simulink model "MF007_MotVltgSVPWM"  (R2022b)
settings: configuration reference "ASW_Configuration_Set_100ms" (kept outside this file)
values from neighbouring files (symbols this model uses):
  MotCtrlModeEnum : value not decoded    [XPSbW_PublicDataType.sldd]
undefined symbols (not defined in the file or in its folder): CalC_MF007_b_ManMotPwmCtrlEna_UL, CalC_MF007_f32_1D3_UL, CalC_MF007_f32_BrdgVoltFbkFilCoeff_UL, CalC_MF007_f32_ManMotPwmACmd_UL, CalC_MF007_f32_ManMotPwmBCmd_UL, CalC_MF007_f32_ManMotPwmCCmd_UL, CalC_MF007_f32_MotBrdgVltg_V, CalC_MF007_f32_MotCtrlPWMPeriodHiLimit_UL, CalC_MF007_f32_MotCtrlPWMPeriodLowLimit_UL, CalC_MF007_f32_MotPWMTimeDelay_s, CalC_MF007_f32_MotTen_UL, CalC_MF007_f32_MotThreeHundredAndFifty_UL, CalC_MF007_f32_MotZeroAgCounter_UL, CalC_MF007_f32_MotZeroAgone_UL, CalC_MF007_f32_MotZeroAgthree_UL, CalC_MF007_f32_MotZeroAgtwo_UL, CalC_MF007_f32_MoyBrdgVoltLo_V, CalC_MF007_f32_Neg1D2_UL, CalC_MF007_f32_Sqrt3D2_UL, CalC_MF007_f32_ZeroAgCalVolt_V, CalC_XPSbW_b_MotTypSeln_UL, CalC_XPSbW_b_MotZeroCalsEn_UL, Con_XPSbW_b_True_UL, Con_XPSbW_f32_1D100_UL, Con_XPSbW_f32_1D2_UL, Con_XPSbW_f32_Deg2Rad_UL, Con_XPSbW_f32_ES003MotAgArbdMax_deg, Con_XPSbW_f32_ES003MotAgArbdMin_deg, Con_XPSbW_f32_ES004MotVelElecFildMax_radps, Con_XPSbW_f32_ES004MotVelElecFildMin_radps, Con_XPSbW_f32_ES008EPSSupplyVltgMax_V, Con_XPSbW_f32_ES008EPSSupplyVltgMin_V, Con_XPSbW_f32_NegOne_UL, Con_XPSbW_f32_One_UL, Con_XPSbW_f32_Sqrt3_UL, Con_XPSbW_f32_Sqrt3D3_UL, Con_XPSbW_f32_Two_UL, Con_XPSbW_f32_Zero_UL, Con_XPSbW_u8_Four_UL, Con_XPSbW_u8_One_UL, Con_XPSbW_u8_Two_UL, Con_XPSbW_u8_Zero_UL
libraries: XpengCHASbWLib x63, simulink x4
(part 1 of 2)
settings Model: DataDictionary=MF007_MotVltgSVPWM.sldd  Creator=donglx1  LastModifiedBy=Xpeng
settings ConfigSetRef: SourceName=ASW_Configuration_Set_100ms

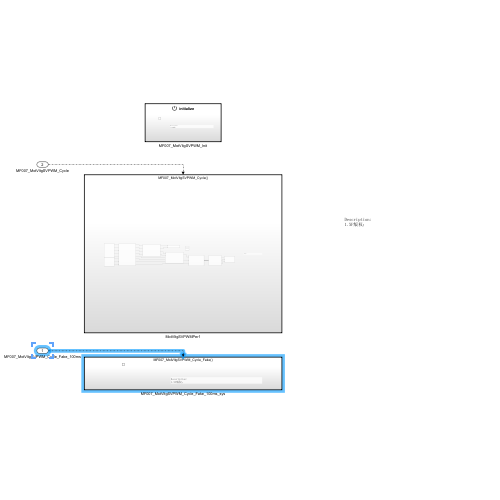
[thumbnail: Simulink's stored preview of the top-level diagram]
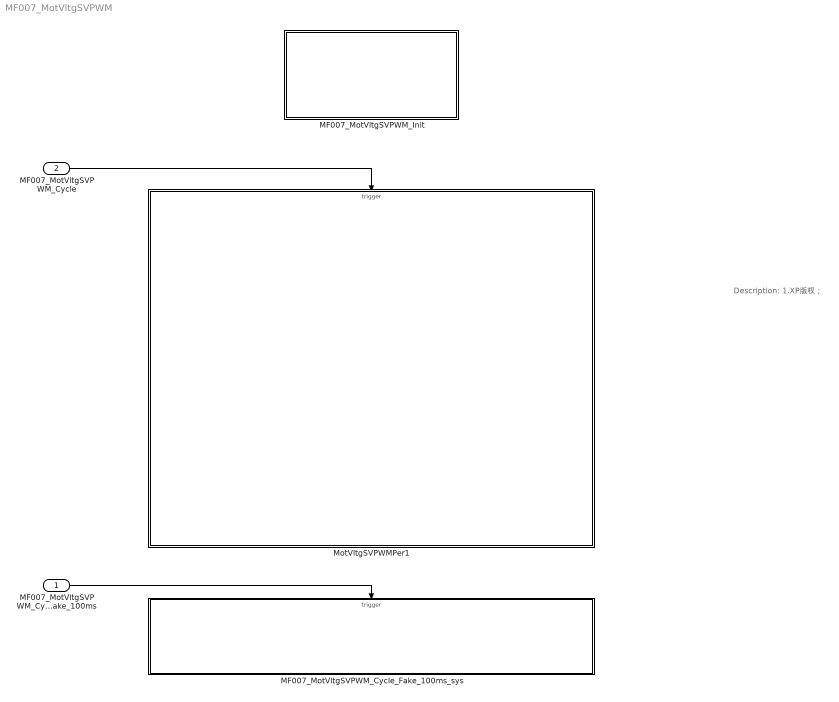
== system MF007_MotVltgSVPWM ==
  note: Description:
      | 1.XP版权；
  MF007_MotVltgSVPWM_Cycle_Fake_100ms : Inport  SampleTime=0.1  OutputFunctionCall=on
  MF007_MotVltgSVPWM_Cycle : Inport  Port=2  SampleTime=0.1  OutputFunctionCall=on
  MF007_MotVltgSVPWM_Cycle_Fake_100ms_sys : Subsystem
  MF007_MotVltgSVPWM_Init : Subsystem
  MotVltgSVPWMPer1 : Subsystem
  wires:
  MF007_MotVltgSVPWM_Cycle_Fake_100ms/1 -> MF007_MotVltgSVPWM_Cycle_Fake_100ms_sys/Trigger
  MF007_MotVltgSVPWM_Cycle/1 -> MotVltgSVPWMPer1/Trigger

== system MF007_MotVltgSVPWM/MF007_MotVltgSVPWM_Cycle_Fake_100ms_sys ==
  note: Description:
      | 1.XP版权；
  MF007_MotVltgSVPWM_Cycle_Fake : TriggerPort  TriggerType=function-call  VariantControl=(inherit)  SampleTimeType=periodic  SampleTime=-1
      settings: AttributesFormatString=|
      | SampleTimeType=%<SampleTimeType>
      | SampleTime=%<SampleTime>

== system MF007_MotVltgSVPWM/MF007_MotVltgSVPWM_Init ==
  note: Description:
      | 1.XP版权；
  MF007_MotVltgSVPWM_Init : EventListener  EventName=reset

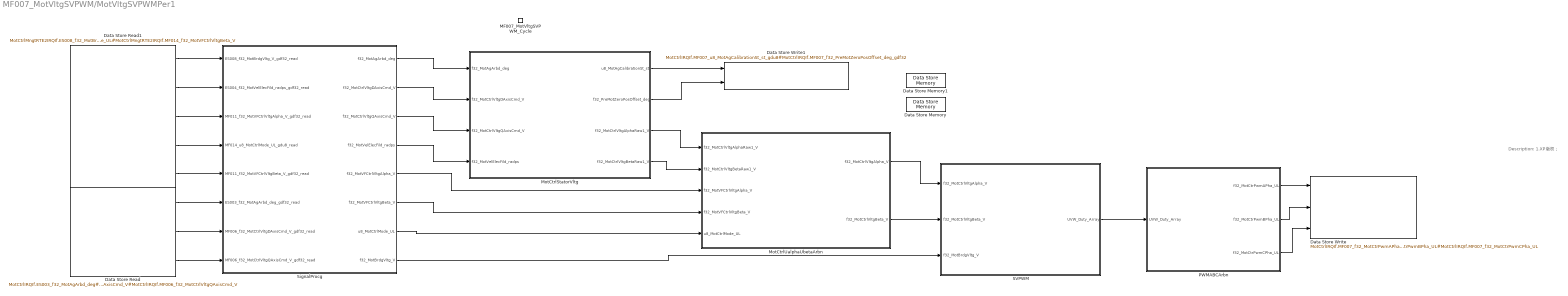
== system MF007_MotVltgSVPWM/MotVltgSVPWMPer1 ==
  note: Description:
      | 1.XP版权；
  MF007_MotVltgSVPWM_Cycle : TriggerPort  TriggerType=function-call  VariantControl=(inherit)  SampleTimeType=periodic  SampleTime=-1
      settings: AttributesFormatString=|
      | SampleTimeType=%<SampleTimeType>
      | SampleTime=%<SampleTime>
  Data Store Memory : XpengCHASbWLib/XpengCHASbWBaseLib/Signal Routing/Data Store Memory  DataStoreName=MotCtrlIRQIf  ReadBeforeWriteMsg=none  WriteAfterWriteMsg=warning  WriteAfterReadMsg=none  InitialValue=0  ShareAcrossModelInstances=off  ShowAdditionalParam=off  OutMin=[]  OutMax=[]  Dimensions=-1  StateMustResolveToSignalObject=on
      settings: SourceProductName=Xpeng CHA SbW Lib  SignalType=auto  DataLogging=off  DataLoggingLimitDataPoints=off  DataLoggingMaxPoints=5000  DataLoggingDecimateData=off  DataLoggingDecimation=2  DataLoggingNameMode=SignalName
  Data Store Memory1 : XpengCHASbWLib/XpengCHASbWBaseLib/Signal Routing/Data Store Memory  DataStoreName=MotCtrlMngtRTE2IRQIf  ReadBeforeWriteMsg=none  WriteAfterWriteMsg=warning  WriteAfterReadMsg=none  InitialValue=0  ShareAcrossModelInstances=off  ShowAdditionalParam=off  OutMin=[]  OutMax=[]  Dimensions=-1  StateMustResolveToSignalObject=on
      settings: SourceProductName=Xpeng CHA SbW Lib  SignalType=auto  DataLogging=off  DataLoggingLimitDataPoints=off  DataLoggingMaxPoints=5000  DataLoggingDecimateData=off  DataLoggingDecimation=2  DataLoggingNameMode=SignalName
  Data Store Read : DataStoreRead  DataStoreName=MotCtrlIRQIf  DataStoreElements=MotCtrlIRQIf.ES003_f32_MotAgArbd_deg#MotCtrlIRQIf.MF006_f32_MotCtrlVltgDAxisCmd_V#MotCtrlIRQIf.MF006_f32_MotCtrlVltgQAxisCmd_V  IndexOptions=Index vector (dialog)  Indices=1  OutputSizes=1
  Data Store Read1 : DataStoreRead  DataStoreName=MotCtrlMngtRTE2IRQIf  DataStoreElements=MotCtrlMngtRTE2IRQIf.ES008_f32_MotBrdgVltg_V#MotCtrlMngtRTE2IRQIf.ES004_f32_MotVelElecFild_radps#MotCtrlMngtRTE2IRQIf.MF014_f32_MotVFCtrlVltgAlpha_V#MotCtrlMngtRTE2IRQIf.MF014_u8_MotCtrlMode_UL#MotCtrlMngtRTE2IRQIf.MF014_f32_MotVFCtrlVltgBeta_V  IndexOptions=Index vector (dialog)  Indices=1  OutputSizes=1
  Data Store Write : DataStoreWrite  DataStoreName=MotCtrlIRQIf  DataStoreElements=MotCtrlIRQIf.MF007_f32_MotCtrPwmAPha_UL#MotCtrlIRQIf.MF007_f32_MotCtrPwmBPha_UL#MotCtrlIRQIf.MF007_f32_MotCtrPwmCPha_UL  IndexOptions=Index vector (dialog)  Indices=1  OutputSizes=1
  Data Store Write1 : DataStoreWrite  DataStoreName=MotCtrlIRQIf  DataStoreElements=MotCtrlIRQIf.MF007_u8_MotAgCalibrationSt_st_gdu8#MotCtrlIRQIf.MF007_f32_PreMotZeroPosOffset_deg_gdf32  IndexOptions=Index vector (dialog)  Indices=1  OutputSizes=1
  MotCtrlStatorVltg : Subsystem
  MotCtrlUalphaUbetaArbn : Subsystem
  PWMABCArbn : Subsystem
  SVPWM : Subsystem
  SignalProcg : Subsystem
  wires:
  SignalProcg/5(f32_MotVFCtrlVltgAlpha_V) -> MotCtrlUalphaUbetaArbn/3(f32_MotVFCtrlVltgAlpha_V)
  MotCtrlUalphaUbetaArbn/1(f32_MotCtrlVltgAlpha_V) -> SVPWM/1(f32_MotCtrlVltgAlpha_V)
  MotCtrlStatorVltg/3(f32_MotCtrlVltgAlphaRaw1_V) -> MotCtrlUalphaUbetaArbn/1(f32_MotCtrlVltgAlphaRaw1_V)
  SignalProcg/4(f32_MotVelElecFild_radps) -> MotCtrlStatorVltg/4(f32_MotVelElecFild_radps)
  SignalProcg/8(f32_MotBrdgVltg_V) -> SVPWM/3(f32_MotBrdgVltg_V)
  SVPWM/1(UVW_Duty_Array) -> PWMABCArbn/1(UVW_Duty_Array)
  MotCtrlStatorVltg/4(f32_MotCtrlVltgBetaRaw1_V) -> MotCtrlUalphaUbetaArbn/2(f32_MotCtrlVltgBetaRaw1_V)
  MotCtrlUalphaUbetaArbn/2(f32_MotCtrlVltgBeta_V) -> SVPWM/2(f32_MotCtrlVltgBeta_V)
  SignalProcg/2(f32_MotCtrlVltgDAxisCmd_V) -> MotCtrlStatorVltg/2(f32_MotCtrlVltgDAxisCmd_V)
  SignalProcg/7(u8_MotCtrlMode_UL) -> MotCtrlUalphaUbetaArbn/5(u8_MotCtrlMode_UL)
  SignalProcg/3(f32_MotCtrlVltgQAxisCmd_V) -> MotCtrlStatorVltg/3(f32_MotCtrlVltgQAxisCmd_V)
  SignalProcg/1(f32_MotAgArbd_deg) -> MotCtrlStatorVltg/1(f32_MotAgArbd_deg)
  SignalProcg/6(f32_MotVFCtrlVltgBeta_V) -> MotCtrlUalphaUbetaArbn/4(f32_MotVFCtrlVltgBeta_V)
  PWMABCArbn/1(f32_MotCtrPwmAPha_UL) -> Data Store Write/1
  PWMABCArbn/2(f32_MotCtrPwmBPha_UL) -> Data Store Write/2
  PWMABCArbn/3(f32_MotCtrPwmCPha_UL) -> Data Store Write/3
  Data Store Read/3 -> SignalProcg/8(MF006_f32_MotCtrlVltgQAxisCmd_V_gdf32_read)
  Data Store Read/2 -> SignalProcg/7(MF006_f32_MotCtrlVltgDAxisCmd_V_gdf32_read)
  Data Store Read/1 -> SignalProcg/6(ES003_f32_MotAgArbd_deg_gdf32_read)
  Data Store Read1/1 -> SignalProcg/1(ES008_f32_MotBrdgVltg_V_gdf32_read)
  Data Store Read1/2 -> SignalProcg/2(ES004_f32_MotVelElecFild_radps_gdf32_read)
  Data Store Read1/3 -> SignalProcg/3(MF011_f32_MotVFCtrlVltgAlpha_V_gdf32_read)
  Data Store Read1/4 -> SignalProcg/4(MF014_u8_MotCtrlMode_UL_gdu8_read)
  Data Store Read1/5 -> SignalProcg/5(MF011_f32_MotVFCtrlVltgBeta_V_gdf32_read)
  MotCtrlStatorVltg/1(u8_MotAgCalibrationSt_st) -> Data Store Write1/1
  MotCtrlStatorVltg/2(f32_PreMotZeroPosOffset_deg) -> Data Store Write1/2

== system MF007_MotVltgSVPWM/MotVltgSVPWMPer1/MotCtrlStatorVltg ==
  note: Description:
      | 1.XP版权；
  f32_MotAgArbd_deg : Inport
  f32_MotCtrlVltgDAxisCmd_V : Inport  Port=2
  f32_MotCtrlVltgQAxisCmd_V : Inport  Port=3
  f32_MotVelElecFild_radps : Inport  Port=4
  Subsystem : Subsystem
  Subsystem1 : Subsystem
  Subsystem2 : Subsystem
  Subsystem4 : Subsystem
  u8_MotAgCalibrationSt_st : Outport
      settings: EnsureOutportIsVirtual=on
  f32_PreMotZeroPosOffset_deg : Outport  Port=2
      settings: EnsureOutportIsVirtual=on
  f32_MotCtrlVltgAlphaRaw1_V : Outport  Port=3
  f32_MotCtrlVltgBetaRaw1_V : Outport  Port=4
  wires:
  f32_MotAgArbd_deg/1 -> Subsystem2/1(f32_MotAgArbd_deg), Subsystem1/1(f32_MotAgArbd_deg)
  Subsystem/1(b_MotZeroAgCalEn_flg) -> Subsystem1/Action
  Subsystem/2(b_MotZeroAgCalDisable_flg) -> Subsystem2/Action
  Subsystem1/1(u8_MotAgCalibrationSt_st) -> u8_MotAgCalibrationSt_st/1
  f32_MotCtrlVltgDAxisCmd_V/1 -> Subsystem2/2(f32_MotCtrlVltgDAxisCmd_V)
  f32_MotCtrlVltgQAxisCmd_V/1 -> Subsystem2/3(f32_MotCtrlVltgQAxisCmd_V)
  f32_MotVelElecFild_radps/1 -> Subsystem2/4(f32_MotVelElecFild_radps)
  Subsystem1/3(f32_MotZeroAgVolUalpha_V) -> Subsystem4/1(f32_MotZeroAgVolUalpha_V)
  Subsystem1/4(f32_MotZeroAgVolubeta_V) -> Subsystem4/2(f32_MotZeroAgVolubeta_V)
  Subsystem2/1(f32_MotCtrlVltgAlphaRaw_V) -> Subsystem4/3(f32_MotCtrlVltgAlphaRaw_V)
  Subsystem2/2(f32_MotCtrlVltgBetaRaw_V) -> Subsystem4/4(f32_MotCtrlVltgBetaRaw_V)
  Subsystem4/2(f32_MotCtrlVltgBetaRaw1_V) -> f32_MotCtrlVltgBetaRaw1_V/1
  Subsystem4/1(f32_MotCtrlVltgAlphaRaw1_V) -> f32_MotCtrlVltgAlphaRaw1_V/1
  Subsystem1/2(f32_PreMotZeroPosOffset_deg) -> f32_PreMotZeroPosOffset_deg/1

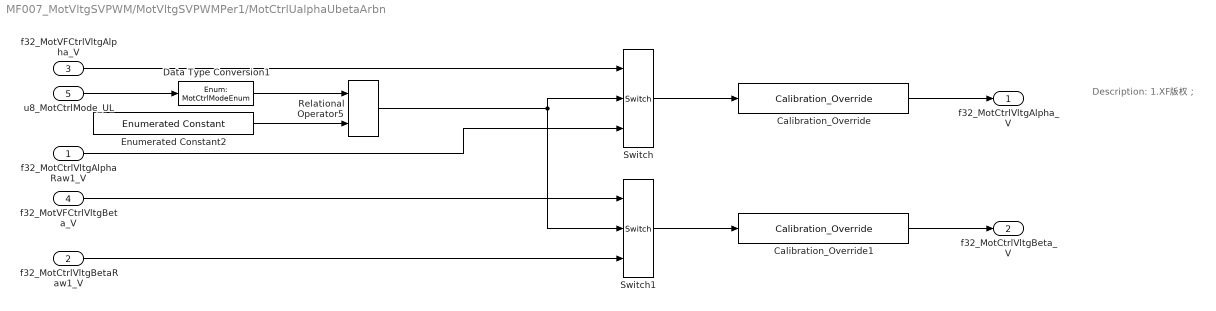
== system MF007_MotVltgSVPWM/MotVltgSVPWMPer1/MotCtrlUalphaUbetaArbn ==
  note: Description:
      | 1.XP版权；
  f32_MotCtrlVltgAlphaRaw1_V : Inport
  f32_MotCtrlVltgBetaRaw1_V : Inport  Port=2
  f32_MotVFCtrlVltgAlpha_V : Inport  Port=3
  f32_MotVFCtrlVltgBeta_V : Inport  Port=4
  u8_MotCtrlMode_UL : Inport  Port=5
  Calibration_Override : XpengCHASbWLib/XpengCHASbWAlgoLib/Signal Routing/Calibration_Override  cal_ovrdflg=CalEn_MF007_b_MotCtrlVltgUalphaEn_UL  cal_ovrdval=CalVal_MF007_f32_MotCtrlVltgUalpha_V
      settings: SourceProductName=Xpeng CHA SbW Lib
      settings: AttributesFormatString=|
      | OvrdEn:%<cal_ovrdflg>
      | OvrdVal:%<cal_ovrdval>
  Calibration_Override1 : XpengCHASbWLib/XpengCHASbWAlgoLib/Signal Routing/Calibration_Override  cal_ovrdflg=CalEn_MF007_b_MotCtrlVltgUbetaEn_UL  cal_ovrdval=CalVal_MF007_f32_MotCtrlVltgUbeta_V
      settings: SourceProductName=Xpeng CHA SbW Lib
      settings: AttributesFormatString=|
      | OvrdEn:%<cal_ovrdflg>
      | OvrdVal:%<cal_ovrdval>
  Data Type Conversion1 : DataTypeConversion  OutDataTypeStr=Enum: MotCtrlModeEnum  SaturateOnIntegerOverflow=off  RndMeth=Floor
  Enumerated Constant2 : simulink/Sources/Enumerated Constant  OutDataTypeStr=Enum: MotCtrlModeEnum  Value=MotCtrlModeEnum.VoltMod  SampleTime=inf
  Relational Operator5 : XpengCHASbWLib/XpengCHASbWBaseLib/Logic Operations/Relational Operator  Operator===  InputSameDT=on  OutDataTypeStr=Inherit: Logical (see Configuration Parameters: Optimization)  SampleTime=-1  RndMeth=Nearest
      settings: SourceProductName=Xpeng CHA SbW Lib
  Switch : XpengCHASbWLib/XpengCHASbWBaseLib/Signal Routing/Switch  Criteria=u2 ~= 0  Threshold=0  InputSameDT=on  OutMin=[]  OutMax=[]  SaturateOnIntegerOverflow=on  SampleTime=-1  AllowDiffInputSizes=off
      settings: AttributesFormatString=%<Criteria>  SourceProductName=Xpeng CHA SbW Lib
  Switch1 : XpengCHASbWLib/XpengCHASbWBaseLib/Signal Routing/Switch  Criteria=u2 ~= 0  Threshold=0  InputSameDT=on  OutMin=[]  OutMax=[]  SaturateOnIntegerOverflow=on  SampleTime=-1  AllowDiffInputSizes=off
      settings: AttributesFormatString=%<Criteria>  SourceProductName=Xpeng CHA SbW Lib
  f32_MotCtrlVltgAlpha_V : Outport
  f32_MotCtrlVltgBeta_V : Outport  Port=2
  wires:
  Switch/1 -> Calibration_Override/1
  Switch1/1 -> Calibration_Override1/1
  u8_MotCtrlMode_UL/1 -> Data Type Conversion1/1
  Enumerated Constant2/1 -> Relational Operator5/2
  Relational Operator5/1 -> Switch/2, Switch1/2
  f32_MotVFCtrlVltgBeta_V/1 -> Switch1/1
  Calibration_Override/1 -> f32_MotCtrlVltgAlpha_V/1
  Calibration_Override1/1 -> f32_MotCtrlVltgBeta_V/1
  f32_MotCtrlVltgAlphaRaw1_V/1 -> Switch/3
  f32_MotCtrlVltgBetaRaw1_V/1 -> Switch1/3
  f32_MotVFCtrlVltgAlpha_V/1 -> Switch/1
  Data Type Conversion1/1 -> Relational Operator5/1

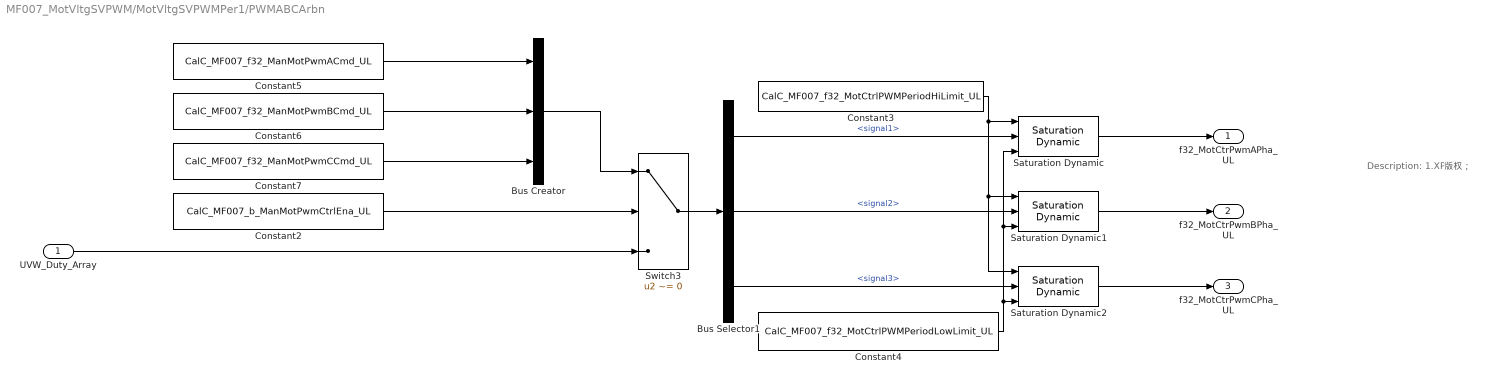
== system MF007_MotVltgSVPWM/MotVltgSVPWMPer1/PWMABCArbn ==
  note: Description:
      | 1.XP版权；
  UVW_Duty_Array : Inport
  Bus Creator : BusCreator  Inputs=3
  Bus Selector1 : BusSelector  OutputSignals=signal1,signal2,signal3
  Constant2 : Constant  Value=CalC_MF007_b_ManMotPwmCtrlEna_UL
  Constant3 : Constant  Value=CalC_MF007_f32_MotCtrlPWMPeriodHiLimit_UL
  Constant4 : Constant  Value=CalC_MF007_f32_MotCtrlPWMPeriodLowLimit_UL
  Constant5 : Constant  Value=CalC_MF007_f32_ManMotPwmACmd_UL
  Constant6 : Constant  Value=CalC_MF007_f32_ManMotPwmBCmd_UL
  Constant7 : Constant  Value=CalC_MF007_f32_ManMotPwmCCmd_UL
  Saturation Dynamic : simulink/Discontinuities/Saturation Dynamic  OutMin=[]  OutMax=[]  OutDataTypeStr=Inherit: Same as second input  OutDataType=fixdt(1, 16)  OutScaling=2^-10  DoSatur=off
  Saturation Dynamic1 : simulink/Discontinuities/Saturation Dynamic  OutMin=[]  OutMax=[]  OutDataTypeStr=Inherit: Same as second input  OutDataType=fixdt(1, 16)  OutScaling=2^-10  DoSatur=off
  Saturation Dynamic2 : simulink/Discontinuities/Saturation Dynamic  OutMin=[]  OutMax=[]  OutDataTypeStr=Inherit: Same as second input  OutDataType=fixdt(1, 16)  OutScaling=2^-10  DoSatur=off
  Switch3 : Switch  Criteria=u2 ~= 0  SaturateOnIntegerOverflow=off  InputSameDT=off
  f32_MotCtrPwmAPha_UL : Outport
      settings: EnsureOutportIsVirtual=on
  f32_MotCtrPwmBPha_UL : Outport  Port=2
      settings: EnsureOutportIsVirtual=on
  f32_MotCtrPwmCPha_UL : Outport  Port=3
      settings: EnsureOutportIsVirtual=on
  wires:
  Switch3/1 -> Bus Selector1/1
  Constant3/1 -> Saturation Dynamic2/1, Saturation Dynamic1/1, Saturation Dynamic/1
  Saturation Dynamic1/1 -> f32_MotCtrPwmBPha_UL/1
  Constant4/1 -> Saturation Dynamic/3, Saturation Dynamic1/3, Saturation Dynamic2/3
  Saturation Dynamic/1 -> f32_MotCtrPwmAPha_UL/1
  Bus Selector1/3 -> Saturation Dynamic2/2  "<signal3>"
  UVW_Duty_Array/1 -> Switch3/3
  Saturation Dynamic2/1 -> f32_MotCtrPwmCPha_UL/1
  Constant5/1 -> Bus Creator/1
  Bus Selector1/1 -> Saturation Dynamic/2  "<signal1>"
  Constant7/1 -> Bus Creator/3
  Bus Selector1/2 -> Saturation Dynamic1/2  "<signal2>"
  Constant2/1 -> Switch3/2
  Constant6/1 -> Bus Creator/2
  Bus Creator/1 -> Switch3/1

== system MF007_MotVltgSVPWM/MotVltgSVPWMPer1/SVPWM ==
  note: Description:
      | 1.XP版权；
  f32_MotCtrlVltgAlpha_V : Inport
  f32_MotCtrlVltgBeta_V : Inport  Port=2
  f32_MotBrdgVltg_V : Inport  Port=3
  OvermodulationProcg : Subsystem
  SectorCal : Subsystem
  XYZ : Subsystem
  XYZ1 : Subsystem
  XYZ2 : Subsystem
  UVW_Duty_Array : Outport  VectorParamsAs1DForOutWhenUnconnected=off
  wires:
  f32_MotCtrlVltgBeta_V/1 -> XYZ/2(f32_MotCtrlVltgBeta_V), SectorCal/2(f32_MotCtrlVltgBeta_V)
  f32_MotCtrlVltgAlpha_V/1 -> XYZ/1(f32_MotCtrlVltgAlpha_V), SectorCal/1(f32_MotCtrlVltgAlpha_V)
  f32_MotBrdgVltg_V/1 -> XYZ/3(f32_MotBrdgVltg_V)
  XYZ/3(Z) -> XYZ1/4(Z)
  XYZ/2(Y) -> XYZ1/3(Y)
  OvermodulationProcg/1(T12_Procg) -> XYZ2/2(T12)
  XYZ/1(X) -> XYZ1/2(X)
  SectorCal/1(u8_MotSector_UL) -> XYZ2/1(u8_MotSector_UL), XYZ1/1(u8_MotSector_UL)
  XYZ2/1(UVW_Duty_Array) -> UVW_Duty_Array/1
  XYZ1/1(T12) -> OvermodulationProcg/1(T12)

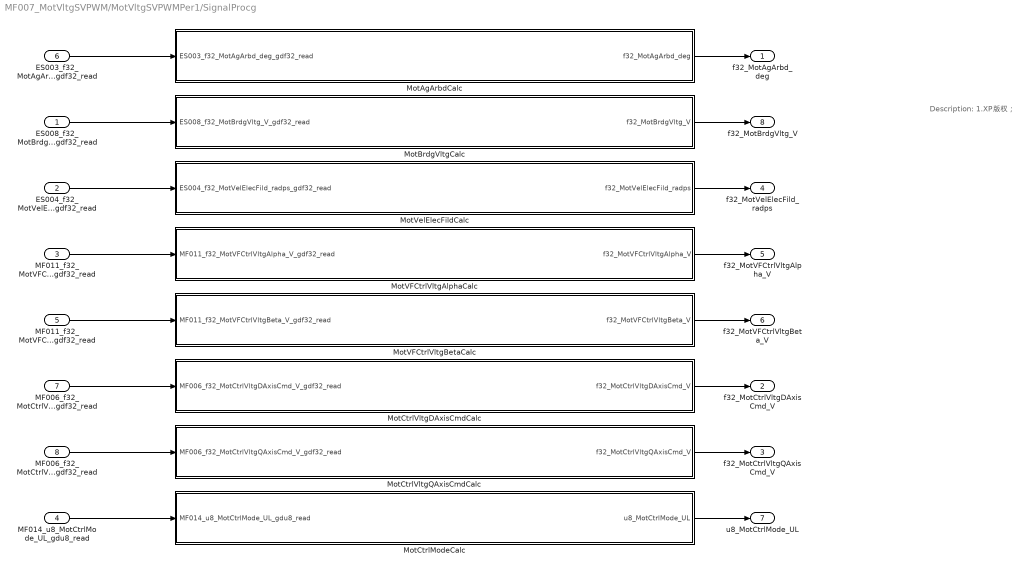
== system MF007_MotVltgSVPWM/MotVltgSVPWMPer1/SignalProcg ==
  note: Description:
      | 1.XP版权；
  ES008_f32_MotBrdgVltg_V_gdf32_read : Inport
  ES004_f32_MotVelElecFild_radps_gdf32_read : Inport  Port=2
  MF011_f32_MotVFCtrlVltgAlpha_V_gdf32_read : Inport  Port=3
  MF014_u8_MotCtrlMode_UL_gdu8_read : Inport  Port=4
  MF011_f32_MotVFCtrlVltgBeta_V_gdf32_read : Inport  Port=5
  ES003_f32_MotAgArbd_deg_gdf32_read : Inport  Port=6
  MF006_f32_MotCtrlVltgDAxisCmd_V_gdf32_read : Inport  Port=7
  MF006_f32_MotCtrlVltgQAxisCmd_V_gdf32_read : Inport  Port=8
  MotAgArbdCalc : Subsystem
  MotBrdgVltgCalc : Subsystem
  MotCtrlModeCalc : Subsystem
  MotCtrlVltgDAxisCmdCalc : Subsystem
  MotCtrlVltgQAxisCmdCalc : Subsystem
  MotVFCtrlVltgAlphaCalc : Subsystem
  MotVFCtrlVltgBetaCalc : Subsystem
  MotVelElecFildCalc : Subsystem
  f32_MotAgArbd_deg : Outport
  f32_MotCtrlVltgDAxisCmd_V : Outport  Port=2
  f32_MotCtrlVltgQAxisCmd_V : Outport  Port=3
  f32_MotVelElecFild_radps : Outport  Port=4
  f32_MotVFCtrlVltgAlpha_V : Outport  Port=5
  f32_MotVFCtrlVltgBeta_V : Outport  Port=6
  u8_MotCtrlMode_UL : Outport  Port=7
  f32_MotBrdgVltg_V : Outport  Port=8
  wires:
  ES004_f32_MotVelElecFild_radps_gdf32_read/1 -> MotVelElecFildCalc/1(ES004_f32_MotVelElecFild_radps_gdf32_read)
  ES008_f32_MotBrdgVltg_V_gdf32_read/1 -> MotBrdgVltgCalc/1(ES008_f32_MotBrdgVltg_V_gdf32_read)
  ES003_f32_MotAgArbd_deg_gdf32_read/1 -> MotAgArbdCalc/1(ES003_f32_MotAgArbd_deg_gdf32_read)
  MotAgArbdCalc/1(f32_MotAgArbd_deg) -> f32_MotAgArbd_deg/1
  MotBrdgVltgCalc/1(f32_MotBrdgVltg_V) -> f32_MotBrdgVltg_V/1
  MotVelElecFildCalc/1(f32_MotVelElecFild_radps) -> f32_MotVelElecFild_radps/1
  MF011_f32_MotVFCtrlVltgAlpha_V_gdf32_read/1 -> MotVFCtrlVltgAlphaCalc/1(MF011_f32_MotVFCtrlVltgAlpha_V_gdf32_read)
  MotVFCtrlVltgAlphaCalc/1(f32_MotVFCtrlVltgAlpha_V) -> f32_MotVFCtrlVltgAlpha_V/1
  MF011_f32_MotVFCtrlVltgBeta_V_gdf32_read/1 -> MotVFCtrlVltgBetaCalc/1(MF011_f32_MotVFCtrlVltgBeta_V_gdf32_read)
  MF006_f32_MotCtrlVltgDAxisCmd_V_gdf32_read/1 -> MotCtrlVltgDAxisCmdCalc/1(MF006_f32_MotCtrlVltgDAxisCmd_V_gdf32_read)
  MF006_f32_MotCtrlVltgQAxisCmd_V_gdf32_read/1 -> MotCtrlVltgQAxisCmdCalc/1(MF006_f32_MotCtrlVltgQAxisCmd_V_gdf32_read)
  MF014_u8_MotCtrlMode_UL_gdu8_read/1 -> MotCtrlModeCalc/1(MF014_u8_MotCtrlMode_UL_gdu8_read)
  MotVFCtrlVltgBetaCalc/1(f32_MotVFCtrlVltgBeta_V) -> f32_MotVFCtrlVltgBeta_V/1
  MotCtrlVltgDAxisCmdCalc/1(f32_MotCtrlVltgDAxisCmd_V) -> f32_MotCtrlVltgDAxisCmd_V/1
  MotCtrlVltgQAxisCmdCalc/1(f32_MotCtrlVltgQAxisCmd_V) -> f32_MotCtrlVltgQAxisCmd_V/1
  MotCtrlModeCalc/1(u8_MotCtrlMode_UL) -> u8_MotCtrlMode_UL/1

== system MF007_MotVltgSVPWM/MotVltgSVPWMPer1/MotCtrlStatorVltg/Subsystem ==
  note: Description:
      | 1.XP版权；
  Constant : Constant  Value=CalC_XPSbW_b_MotZeroCalsEn_UL
  If : If  IfExpression=u1 == 1
  b_MotZeroAgCalEn_flg : Outport
  b_MotZeroAgCalDisable_flg : Outport  Port=2
  wires:
  Constant/1 -> If/1
  If/2 -> b_MotZeroAgCalDisable_flg/1
  If/1 -> b_MotZeroAgCalEn_flg/1

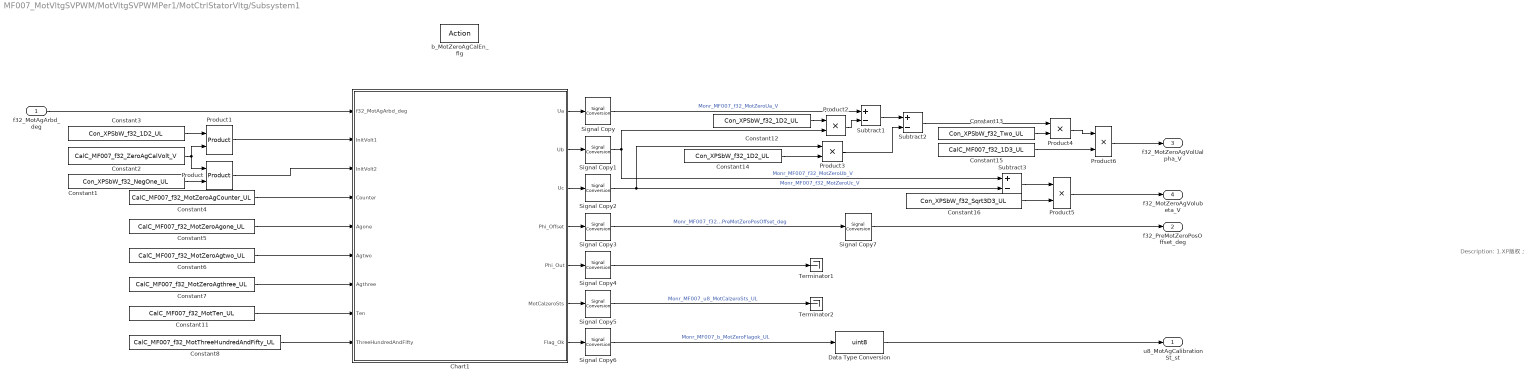
== system MF007_MotVltgSVPWM/MotVltgSVPWMPer1/MotCtrlStatorVltg/Subsystem1 ==
  note: Description:
      | 1.XP版权；
  f32_MotAgArbd_deg : Inport
  b_MotZeroAgCalEn_flg : ActionPort  ActionPortLabel=if(u1 == 1)
  Chart1 : Stateflow chart  TreatAsAtomicUnit=on
      settings: PortSchema="{\"entries\":[{\"content\":{\"sides\":[{\"content\":{\"connectorIds\":[\"In1\",\"In2\",\"In3\",\"In4\",\"In5\",\"In7\",\"In6\",\"In8\",\"In9\"]},\"type\":\"ConnectorPlacement.EquallySpacedRectSide\",\"uuid\":\"c0b776fd-f9c3-46a3-bcf2-78277c181056\"},{\"content\":{\"connectorIds\":[\"Out1\",\"Out2\",\"Out3\",\"Out4\",\"Out6\",\"Out7\",\"Out5\"],\"side\":\"RIGHT\"},\"type\":\"ConnectorPlacement.EquallySpacedRectSide\",\"uuid\":\"faec2a9b-d18f-4659-a1ec-eeaa302fe436\"},{\"content\":{\"connectorIds\":[],\"side\":\"TOP\"},\"type\":\"ConnectorPlacement.EquallySpacedRectSide\",\"uuid\":\"ae3a4ef0-e647-4d80-9ccb-63a892ad0e59\"}]},\"type\":\"ConnectorPlacement.EquallySpacedConnector\",\"uuid\":\"88ddbb7a-b53a-4e2b-831c-a44bbab1e19b\"}],\"packageUris\":[\"http://schema.mathworks.com/mf0/Connector/R2020b\"],\"version\":\"1.0\"}"
  Constant1 : Constant  Value=Con_XPSbW_f32_NegOne_UL
  Constant11 : Constant  Value=CalC_MF007_f32_MotTen_UL
  Constant12 : Constant  Value=Con_XPSbW_f32_1D2_UL  OutDataTypeStr=single
  Constant13 : Constant  Value=Con_XPSbW_f32_Two_UL  OutDataTypeStr=single
  Constant14 : Constant  Value=Con_XPSbW_f32_1D2_UL  OutDataTypeStr=single
  Constant15 : Constant  Value=CalC_MF007_f32_1D3_UL  OutDataTypeStr=single
  Constant16 : Constant  Value=Con_XPSbW_f32_Sqrt3D3_UL
  Constant2 : Constant  Value=CalC_MF007_f32_ZeroAgCalVolt_V  OutDataTypeStr=single
  Constant3 : Constant  Value=Con_XPSbW_f32_1D2_UL
  Constant4 : Constant  Value=CalC_MF007_f32_MotZeroAgCounter_UL
  Constant5 : Constant  Value=CalC_MF007_f32_MotZeroAgone_UL
  Constant6 : Constant  Value=CalC_MF007_f32_MotZeroAgtwo_UL
  Constant7 : Constant  Value=CalC_MF007_f32_MotZeroAgthree_UL
  Constant8 : Constant  Value=CalC_MF007_f32_MotThreeHundredAndFifty_UL
  Data Type Conversion : DataTypeConversion  OutDataTypeStr=uint8  SaturateOnIntegerOverflow=off  RndMeth=Floor
  Product : XpengCHASbWLib/XpengCHASbWBaseLib/Math Operations/Product  Inputs=2  Multiplication=Element-wise(.*)  CollapseDim=1  OutMin=[]  OutMax=[]  RndMeth=Zero  SaturateOnIntegerOverflow=on  SampleTime=-1
      settings: SourceProductName=Xpeng CHA SbW Lib
  Product1 : XpengCHASbWLib/XpengCHASbWBaseLib/Math Operations/Product  Inputs=2  Multiplication=Element-wise(.*)  CollapseDim=1  OutMin=[]  OutMax=[]  RndMeth=Zero  SaturateOnIntegerOverflow=on  SampleTime=-1
      settings: SourceProductName=Xpeng CHA SbW Lib
  Product{2..6} (5 alike) : Product
  Signal Copy{,1..7} (8 alike) : SignalConversion  OverrideOpt=off
  Subtract1 : Sum  Inputs=+-
  Subtract2 : Sum  Inputs=+-
  Subtract3 : Sum  Inputs=+-
  Terminator1 : Terminator
  Terminator2 : Terminator
  u8_MotAgCalibrationSt_st : Outport
  f32_PreMotZeroPosOffset_deg : Outport  Port=2
      settings: EnsureOutportIsVirtual=on
  f32_MotZeroAgVolUalpha_V : Outport  Port=3  VectorParamsAs1DForOutWhenUnconnected=off
  f32_MotZeroAgVolubeta_V : Outport  Port=4  VectorParamsAs1DForOutWhenUnconnected=off
  wires:
  Constant7/1 -> Chart1/6(Agthree)
  Product1/1 -> Chart1/2(InitVolt1)
  Constant1/1 -> Product/2
  Chart1/1(Ua) -> Signal Copy/1
  Constant4/1 -> Chart1/4(Counter)
  Constant6/1 -> Chart1/7(Agtwo)
  Signal Copy2/1 -> Subtract3/2, Product3/1  "Monr_MF007_f32_MotZeroUc_V"
  Constant2/1 -> Product/1, Product1/2
  Product/1 -> Chart1/3(InitVolt2)
  Constant5/1 -> Chart1/5(Agone)
  f32_MotAgArbd_deg/1 -> Chart1/1(f32_MotAgArbd_deg)
  Constant3/1 -> Product1/1
  Signal Copy3/1 -> Signal Copy7/1  "Monr_MF007_f32_PreMotZeroPosOffset_deg"
  Signal Copy1/1 -> Product2/2, Subtract3/1  "Monr_MF007_f32_MotZeroUb_V"
  Product6/1 -> f32_MotZeroAgVolUalpha_V/1
  Product5/1 -> f32_MotZeroAgVolubeta_V/1
  Signal Copy6/1 -> Data Type Conversion/1  "Monr_MF007_b_MotZeroFlagok_UL"
  Data Type Conversion/1 -> u8_MotAgCalibrationSt_st/1
  Constant11/1 -> Chart1/8(Ten)
  Constant12/1 -> Product2/1
  Product2/1 -> Subtract1/2
  Constant14/1 -> Product3/2
  Subtract1/1 -> Subtract2/1
  Product3/1 -> Subtract2/2
  Subtract2/1 -> Product4/1
  Constant13/1 -> Product4/2
  Product4/1 -> Product6/1
  Constant15/1 -> Product6/2
  Constant16/1 -> Product5/2
  Subtract3/1 -> Product5/1
  Signal Copy5/1 -> Terminator2/1  "Monr_MF007_u8_MotCalzeroSts_UL"
  Signal Copy/1 -> Subtract1/1  "Monr_MF007_f32_MotZeroUa_V"
  Chart1/2(Ub) -> Signal Copy1/1
  Chart1/3(Uc) -> Signal Copy2/1
  Chart1/4(Phi_Offset) -> Signal Copy3/1
  Chart1/7(MotCalzeroSts) -> Signal Copy5/1
  Chart1/6(Phi_Out) -> Signal Copy4/1
  Chart1/5(Flag_Ok) -> Signal Copy6/1
  Signal Copy7/1 -> f32_PreMotZeroPosOffset_deg/1
  Constant8/1 -> Chart1/9(ThreeHundredAndFifty)
  Signal Copy4/1 -> Terminator1/1

== system MF007_MotVltgSVPWM/MotVltgSVPWMPer1/MotCtrlStatorVltg/Subsystem2 ==
  note: Description:
      | 1.XP版权；
  f32_MotAgArbd_deg : Inport
  f32_MotCtrlVltgDAxisCmd_V : Inport  Port=2
  f32_MotCtrlVltgQAxisCmd_V : Inport  Port=3
  f32_MotVelElecFild_radps : Inport  Port=4
  b_MotZeroAgCalDisable_flg : ActionPort  ActionPortLabel=else
  Subsystem : Subsystem
  Subsystem1 : Subsystem
  Subsystem2 : Subsystem
  Subsystem3 : Subsystem
  Subsystem4 : Subsystem
  f32_MotCtrlVltgAlphaRaw_V : Outport
  f32_MotCtrlVltgBetaRaw_V : Outport  Port=2
  wires:
  f32_MotAgArbd_deg/1 -> Subsystem/1(f32_MotAgArbd_deg)
  f32_MotCtrlVltgDAxisCmd_V/1 -> Subsystem/2(f32_MotCtrlVltgDAxisCmd_V)
  f32_MotCtrlVltgQAxisCmd_V/1 -> Subsystem/3(f32_MotCtrlVltgQAxisCmd_V)
  f32_MotVelElecFild_radps/1 -> Subsystem/4(f32_MotVelElecFild_radps)
  Subsystem/1(f32_MotCtrlVltgAlpha_V) -> Subsystem3/1(f32_MotCtrlVltgAlphaRaw_V), Subsystem2/1(f32_MotCtrlVltgAlphaRaw_V)
  Subsystem/2(f32_MotCtrlVltgBeta_V) -> Subsystem2/2(f32_MotCtrlVltgBetaRaw_V), Subsystem3/2(f32_MotCtrlVltgBetaRaw_V)
  Subsystem1/1(StarMotor) -> Subsystem2/Action
  Subsystem1/2(DeltaMotor) -> Subsystem3/Action
  Subsystem2/1(f32_StarMotCtrlVltgAlpha_V) -> Subsystem4/1(f32_StarMotCtrlVltgAlpha_V)
  Subsystem2/2(f32_StarMotCtrlVltgBeta_V) -> Subsystem4/2(f32_StarMotCtrlVltgBeta_V)
  Subsystem3/1(f32_DeltaMotCtrlVltgAlpha_V) -> Subsystem4/3(f32_DeltaMotCtrlVltgAlpha_V)
  Subsystem3/2(f32_DeltaMotCtrlVltgBeta_V) -> Subsystem4/4(f32_DeltaMotCtrlVltgBeta_V)
  Subsystem4/1(f32_MotCtrlVltgAlphaRaw_V) -> f32_MotCtrlVltgAlphaRaw_V/1
  Subsystem4/2(f32_MotCtrlVltgBetaRaw_V) -> f32_MotCtrlVltgBetaRaw_V/1

== system MF007_MotVltgSVPWM/MotVltgSVPWMPer1/MotCtrlStatorVltg/Subsystem4 ==
  note: Description:
      | 1.XP版权；
  f32_MotZeroAgVolUalpha_V : Inport
  f32_MotZeroAgVolubeta_V : Inport  Port=2
  f32_MotCtrlVltgAlphaRaw_V : Inport  Port=3
  f32_MotCtrlVltgBetaRaw_V : Inport  Port=4
  Merge : Merge
  Merge1 : Merge
  f32_MotCtrlVltgAlphaRaw1_V : Outport
  f32_MotCtrlVltgBetaRaw1_V : Outport  Port=2
  wires:
  f32_MotZeroAgVolUalpha_V/1 -> Merge/1
  f32_MotCtrlVltgAlphaRaw_V/1 -> Merge/2
  Merge/1 -> f32_MotCtrlVltgAlphaRaw1_V/1
  f32_MotZeroAgVolubeta_V/1 -> Merge1/1
  f32_MotCtrlVltgBetaRaw_V/1 -> Merge1/2
  Merge1/1 -> f32_MotCtrlVltgBetaRaw1_V/1

== system MF007_MotVltgSVPWM/MotVltgSVPWMPer1/SVPWM/OvermodulationProcg ==
  note: Description:
      | 1.XP版权；
  T12 : Inport
  Add : Sum
  Bus Creator6 : BusCreator  Inputs=2
  Bus Selector : BusSelector  OutputSignals=signal1,signal2
  Constant1 : Constant  Value=Con_XPSbW_f32_One_UL
  DIV : XpengCHASbWLib/XpengCHASbWBaseLib/Math Operations/DIV  MinRange=single(1e-6)
      settings: SourceProductName=Xpeng CHA SbW Lib
  DIV1 : XpengCHASbWLib/XpengCHASbWBaseLib/Math Operations/DIV  MinRange=single(1e-6)
      settings: SourceProductName=Xpeng CHA SbW Lib
  Relational Operator : RelationalOperator  Operator=>  RndMeth=Simplest  InputSameDT=off
  Switch : XpengCHASbWLib/XpengCHASbWBaseLib/Signal Routing/Switch  Criteria=u2 ~= 0  Threshold=0  InputSameDT=on  OutMin=[]  OutMax=[]  SaturateOnIntegerOverflow=on  SampleTime=-1  AllowDiffInputSizes=off
      settings: AttributesFormatString=%<Criteria>  SourceProductName=Xpeng CHA SbW Lib
  T12_Procg : Outport
  wires:
  DIV1/1 -> Bus Creator6/2
  Bus Creator6/1 -> Switch/1
  Add/1 -> DIV/2, DIV1/2, Relational Operator/1
  T12/1 -> Bus Selector/1, Switch/3
  Bus Selector/2 -> Add/2, DIV1/1  "<signal2>"
  DIV/1 -> Bus Creator6/1
  Bus Selector/1 -> Add/1, DIV/1  "<signal1>"
  Switch/1 -> T12_Procg/1
  Constant1/1 -> Relational Operator/2
  Relational Operator/1 -> Switch/2

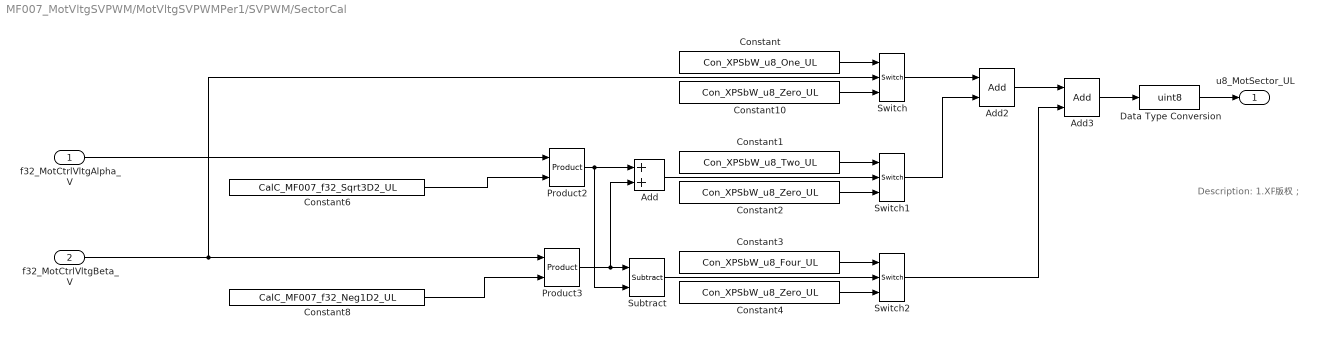
== system MF007_MotVltgSVPWM/MotVltgSVPWMPer1/SVPWM/SectorCal ==
  note: Description:
      | 1.XP版权；
  f32_MotCtrlVltgAlpha_V : Inport
  f32_MotCtrlVltgBeta_V : Inport  Port=2
  Add : Sum
  Add2 : XpengCHASbWLib/XpengCHASbWBaseLib/Math Operations/Add  Inputs=++  CollapseDim=1  OutMin=[]  OutMax=[]  SampleTime=-1
      settings: SourceProductName=Xpeng CHA SbW Lib
  Add3 : XpengCHASbWLib/XpengCHASbWBaseLib/Math Operations/Add  Inputs=++  CollapseDim=1  OutMin=[]  OutMax=[]  SampleTime=-1
      settings: SourceProductName=Xpeng CHA SbW Lib
  Constant : Constant  Value=Con_XPSbW_u8_One_UL  OutDataTypeStr=single
  Constant1 : Constant  Value=Con_XPSbW_u8_Two_UL  OutDataTypeStr=single
  Constant10 : Constant  Value=Con_XPSbW_u8_Zero_UL  OutDataTypeStr=single
  Constant2 : Constant  Value=Con_XPSbW_u8_Zero_UL  OutDataTypeStr=single
  Constant3 : Constant  Value=Con_XPSbW_u8_Four_UL  OutDataTypeStr=single
  Constant4 : Constant  Value=Con_XPSbW_u8_Zero_UL  OutDataTypeStr=single
  Constant6 : Constant  Value=CalC_MF007_f32_Sqrt3D2_UL
  Constant8 : Constant  Value=CalC_MF007_f32_Neg1D2_UL
  Data Type Conversion : DataTypeConversion  OutDataTypeStr=uint8  SaturateOnIntegerOverflow=off  RndMeth=Floor
  Product2 : XpengCHASbWLib/XpengCHASbWBaseLib/Math Operations/Product  Inputs=2  Multiplication=Element-wise(.*)  CollapseDim=1  OutMin=[]  OutMax=[]  RndMeth=Zero  SaturateOnIntegerOverflow=on  SampleTime=-1
      settings: SourceProductName=Xpeng CHA SbW Lib
  Product3 : XpengCHASbWLib/XpengCHASbWBaseLib/Math Operations/Product  Inputs=2  Multiplication=Element-wise(.*)  CollapseDim=1  OutMin=[]  OutMax=[]  RndMeth=Zero  SaturateOnIntegerOverflow=on  SampleTime=-1
      settings: SourceProductName=Xpeng CHA SbW Lib
  Subtract : XpengCHASbWLib/XpengCHASbWBaseLib/Math Operations/Subtract  Inputs=+-  CollapseDim=1  OutMin=[]  OutMax=[]  SampleTime=-1
      settings: SourceProductName=Xpeng CHA SbW Lib
  Switch : XpengCHASbWLib/XpengCHASbWBaseLib/Signal Routing/Switch  Criteria=u2 > Threshold  Threshold=0  InputSameDT=on  OutMin=[]  OutMax=[]  SaturateOnIntegerOverflow=on  SampleTime=-1  AllowDiffInputSizes=off
      settings: AttributesFormatString=%<Criteria>  SourceProductName=Xpeng CHA SbW Lib
  Switch1 : XpengCHASbWLib/XpengCHASbWBaseLib/Signal Routing/Switch  Criteria=u2 > Threshold  Threshold=0  InputSameDT=on  OutMin=[]  OutMax=[]  SaturateOnIntegerOverflow=on  SampleTime=-1  AllowDiffInputSizes=off
      settings: AttributesFormatString=%<Criteria>  SourceProductName=Xpeng CHA SbW Lib
  Switch2 : XpengCHASbWLib/XpengCHASbWBaseLib/Signal Routing/Switch  Criteria=u2 > Threshold  Threshold=0  InputSameDT=on  OutMin=[]  OutMax=[]  SaturateOnIntegerOverflow=on  SampleTime=-1  AllowDiffInputSizes=off
      settings: AttributesFormatString=%<Criteria>  SourceProductName=Xpeng CHA SbW Lib
  u8_MotSector_UL : Outport
  wires:
  Constant/1 -> Switch/1
  f32_MotCtrlVltgAlpha_V/1 -> Product2/1
  Constant10/1 -> Switch/3
  f32_MotCtrlVltgBeta_V/1 -> Switch/2, Product3/1
  Product2/1 -> Subtract/2, Add/1
  Product3/1 -> Add/2, Subtract/1
  Constant1/1 -> Switch1/1
  Constant2/1 -> Switch1/3
  Add/1 -> Switch1/2
  Constant3/1 -> Switch2/1
  Subtract/1 -> Switch2/2
  Add3/1 -> Data Type Conversion/1
  Constant6/1 -> Product2/2
  Constant8/1 -> Product3/2
  Constant4/1 -> Switch2/3
  Switch/1 -> Add2/1
  Switch1/1 -> Add2/2
  Add2/1 -> Add3/1
  Switch2/1 -> Add3/2
  Data Type Conversion/1 -> u8_MotSector_UL/1

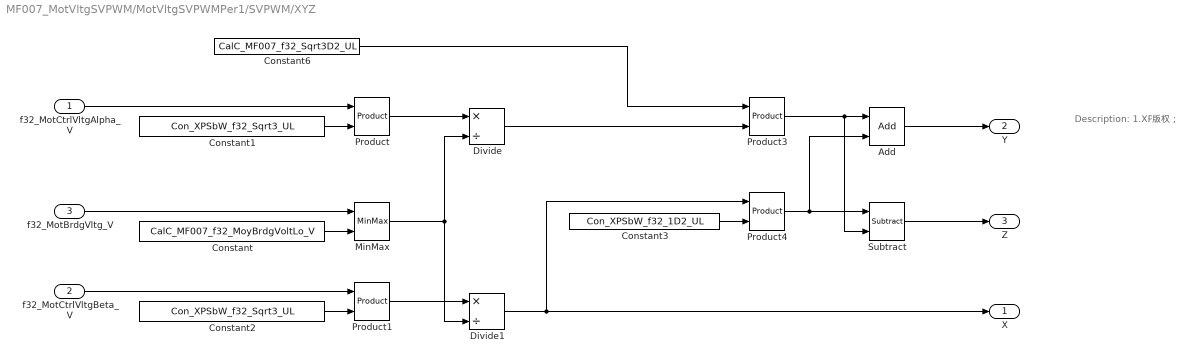
== system MF007_MotVltgSVPWM/MotVltgSVPWMPer1/SVPWM/XYZ ==
  note: Description:
      | 1.XP版权；
  f32_MotCtrlVltgAlpha_V : Inport
  f32_MotCtrlVltgBeta_V : Inport  Port=2
  f32_MotBrdgVltg_V : Inport  Port=3
  Add : XpengCHASbWLib/XpengCHASbWBaseLib/Math Operations/Add  Inputs=++  CollapseDim=1  OutMin=[]  OutMax=[]  SampleTime=-1
      settings: SourceProductName=Xpeng CHA SbW Lib
  Constant : Constant  Value=CalC_MF007_f32_MoyBrdgVoltLo_V  OutDataTypeStr=single
  Constant1 : Constant  Value=Con_XPSbW_f32_Sqrt3_UL  OutDataTypeStr=single
  Constant2 : Constant  Value=Con_XPSbW_f32_Sqrt3_UL  OutDataTypeStr=single
  Constant3 : Constant  Value=Con_XPSbW_f32_1D2_UL
  Constant6 : Constant  Value=CalC_MF007_f32_Sqrt3D2_UL
  Divide : Product  Inputs=*/
  Divide1 : Product  Inputs=*/
  MinMax : XpengCHASbWLib/XpengCHASbWBaseLib/Math Operations/MinMax  Function=max  Inputs=2  InputSameDT=on  OutMin=[]  OutMax=[]  SaturateOnIntegerOverflow=on  SampleTime=-1
      settings: SourceProductName=Xpeng CHA SbW Lib
  Product{,1,3..4} (4 alike) : XpengCHASbWLib/XpengCHASbWBaseLib/Math Operations/Product  Inputs=2  Multiplication=Element-wise(.*)  CollapseDim=1  OutMin=[]  OutMax=[]  RndMeth=Zero  SaturateOnIntegerOverflow=on  SampleTime=-1
      settings: SourceProductName=Xpeng CHA SbW Lib
  Subtract : XpengCHASbWLib/XpengCHASbWBaseLib/Math Operations/Subtract  Inputs=+-  CollapseDim=1  OutMin=[]  OutMax=[]  SampleTime=-1
      settings: SourceProductName=Xpeng CHA SbW Lib
  X : Outport
  Y : Outport  Port=2
  Z : Outport  Port=3
  wires:
  f32_MotCtrlVltgAlpha_V/1 -> Product/1
  Product/1 -> Divide/1
  f32_MotBrdgVltg_V/1 -> MinMax/1
  f32_MotCtrlVltgBeta_V/1 -> Product1/1
  Product1/1 -> Divide1/1
  Divide1/1 -> X/1, Product4/1
  Divide/1 -> Product3/2
  Product3/1 -> Add/1, Subtract/2
  Product4/1 -> Add/2, Subtract/1
  Add/1 -> Y/1
  Subtract/1 -> Z/1
  MinMax/1 -> Divide1/2, Divide/2
  Constant/1 -> MinMax/2
  Constant1/1 -> Product/2
  Constant2/1 -> Product1/2
  Constant6/1 -> Product3/1
  Constant3/1 -> Product4/2

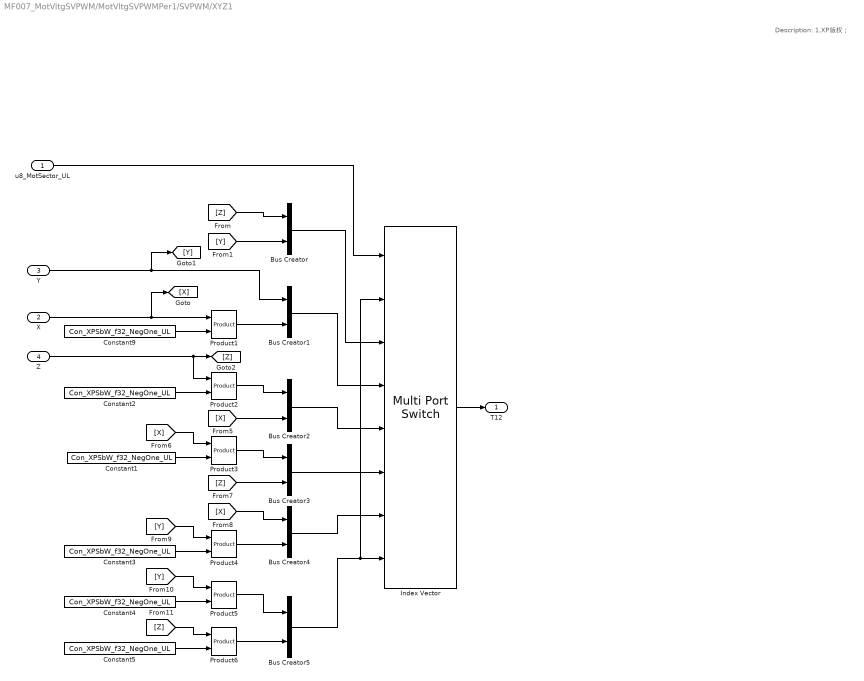
== system MF007_MotVltgSVPWM/MotVltgSVPWMPer1/SVPWM/XYZ1 ==
  note: Description:
      | 1.XP版权；
  u8_MotSector_UL : Inport
  X : Inport  Port=2
  Y : Inport  Port=3
  Z : Inport  Port=4
  Bus Creator{,1..5} (6 alike) : BusCreator  Inputs=2
  Constant{1..5,9} (6 alike) : Constant  Value=Con_XPSbW_f32_NegOne_UL
  Index Vector : MultiPortSwitch  DataPortOrder=Zero-based contiguous  Inputs=7  DataPortIndices={1,2,3,4,5,6}  DiagnosticForDefault=None  zeroidx=on  SaturateOnIntegerOverflow=off  InputSameDT=off
  Product{1..6} (6 alike) : XpengCHASbWLib/XpengCHASbWBaseLib/Math Operations/Product  Inputs=2  Multiplication=Element-wise(.*)  CollapseDim=1  OutMin=[]  OutMax=[]  RndMeth=Zero  SaturateOnIntegerOverflow=on  SampleTime=-1
      settings: SourceProductName=Xpeng CHA SbW Lib
  T12 : Outport
  wires:
  Index Vector/1 -> T12/1
  X/1 -> Product1/1, [X]
  Constant3/1 -> Product4/2
  [Z] -> Bus Creator3/2
  Constant2/1 -> Product2/2
  Constant1/1 -> Product3/2
  Constant9/1 -> Product1/2
  [X] -> Product3/1
  Z/1 -> [Z], Product2/1
  [Y] -> Product4/1
  Y/1 -> Bus Creator1/1, [Y]
  [Y] -> Product5/1
  [X] -> Bus Creator2/2
  [Z] -> Product6/1
  Constant4/1 -> Product5/2
  Constant5/1 -> Product6/2
  [Z] -> Bus Creator/1
  [Y] -> Bus Creator/2
  Product1/1 -> Bus Creator1/2
  Product2/1 -> Bus Creator2/1
  Product3/1 -> Bus Creator3/1
  [X] -> Bus Creator4/1
  Product6/1 -> Bus Creator5/2
  Product4/1 -> Bus Creator4/2
  Product5/1 -> Bus Creator5/1
  u8_MotSector_UL/1 -> Index Vector/1
  Bus Creator/1 -> Index Vector/3
  Bus Creator1/1 -> Index Vector/4
  Bus Creator2/1 -> Index Vector/5
  Bus Creator3/1 -> Index Vector/6
  Bus Creator4/1 -> Index Vector/7
  Bus Creator5/1 -> Index Vector/2, Index Vector/8

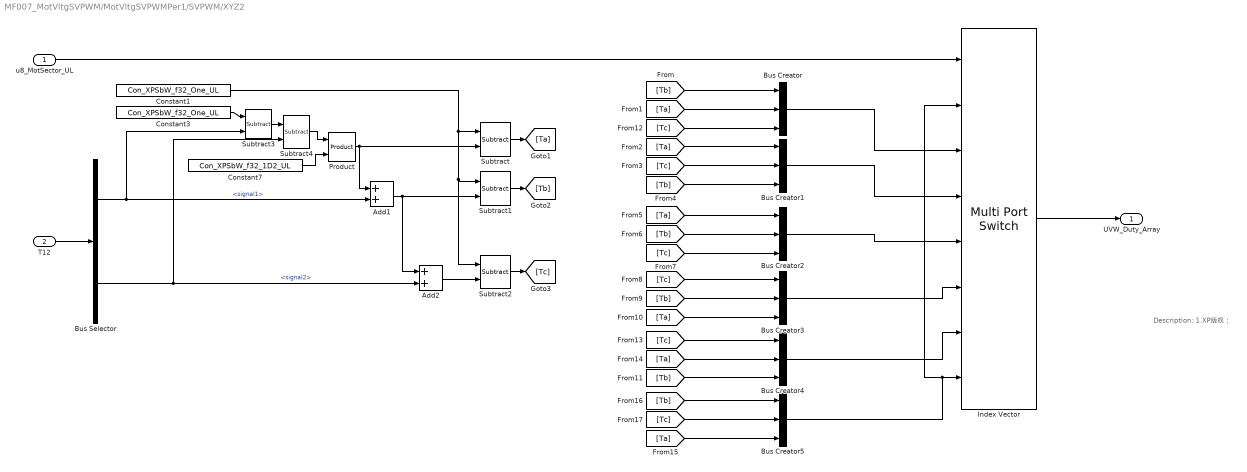
== system MF007_MotVltgSVPWM/MotVltgSVPWMPer1/SVPWM/XYZ2 ==
  note: Description:
      | 1.XP版权；
  u8_MotSector_UL : Inport
  T12 : Inport  Port=2
  Add1 : Sum
  Add2 : Sum
  Bus Creator{,1..5} (6 alike) : BusCreator  Inputs=3
  Bus Selector : BusSelector  OutputSignals=signal1,signal2
  Constant1 : Constant  Value=Con_XPSbW_f32_One_UL
  Constant3 : Constant  Value=Con_XPSbW_f32_One_UL
  Constant7 : Constant  Value=Con_XPSbW_f32_1D2_UL
  Index Vector : MultiPortSwitch  DataPortOrder=Zero-based contiguous  Inputs=7  DataPortIndices={1,2,3,4,5,6}  DiagnosticForDefault=None  zeroidx=on  SaturateOnIntegerOverflow=off  InputSameDT=off
  Product : XpengCHASbWLib/XpengCHASbWBaseLib/Math Operations/Product  Inputs=2  Multiplication=Element-wise(.*)  CollapseDim=1  OutMin=[]  OutMax=[]  RndMeth=Zero  SaturateOnIntegerOverflow=on  SampleTime=-1
      settings: SourceProductName=Xpeng CHA SbW Lib
  Subtract{,1..4} (5 alike) : XpengCHASbWLib/XpengCHASbWBaseLib/Math Operations/Subtract  Inputs=+-  CollapseDim=1  OutMin=[]  OutMax=[]  SampleTime=-1
      settings: SourceProductName=Xpeng CHA SbW Lib
  UVW_Duty_Array : Outport
  wires:
  Index Vector/1 -> UVW_Duty_Array/1
  [Ta] -> Bus Creator/2
  [Tb] -> Bus Creator/1
  u8_MotSector_UL/1 -> Index Vector/1
  [Tc] -> Bus Creator/3
  [Tc] -> Bus Creator1/2
  [Ta] -> Bus Creator1/1
  [Tb] -> Bus Creator1/3
  [Tb] -> Bus Creator2/2
  [Ta] -> Bus Creator2/1
  [Tc] -> Bus Creator2/3
  [Tb] -> Bus Creator3/2
  [Tc] -> Bus Creator3/1
  [Ta] -> Bus Creator3/3
  [Ta] -> Bus Creator4/2
  [Tc] -> Bus Creator4/1
  [Tb] -> Bus Creator4/3
  [Tc] -> Bus Creator5/2
  [Tb] -> Bus Creator5/1
  [Ta] -> Bus Creator5/3
  Add1/1 -> Subtract1/2, Add2/1
  T12/1 -> Bus Selector/1
  Bus Selector/2 -> Subtract4/2, Add2/2  "<signal2>"
  Constant3/1 -> Subtract3/1
  Subtract2/1 -> [Tc]
  Subtract3/1 -> Subtract4/1
  Bus Selector/1 -> Add1/2, Subtract3/2  "<signal1>"
  Product/1 -> Subtract/2, Add1/1
  Constant1/1 -> Subtract1/1, Subtract2/1, Subtract/1
  Subtract/1 -> [Ta]
  Add2/1 -> Subtract2/2
  Subtract1/1 -> [Tb]
  Constant7/1 -> Product/2
  Subtract4/1 -> Product/1
  Bus Creator/1 -> Index Vector/3
  Bus Creator1/1 -> Index Vector/4
  Bus Creator2/1 -> Index Vector/5
  Bus Creator3/1 -> Index Vector/6
  Bus Creator4/1 -> Index Vector/7
  Bus Creator5/1 -> Index Vector/2, Index Vector/8

== system MF007_MotVltgSVPWM/MotVltgSVPWMPer1/SignalProcg/MotAgArbdCalc ==
  note: Description:
      | 1.XP版权；
  ES003_f32_MotAgArbd_deg_gdf32_read : Inport
  Constant : Constant  Value=Con_XPSbW_f32_ES003MotAgArbdMax_deg
  Constant1 : Constant  Value=Con_XPSbW_f32_ES003MotAgArbdMin_deg
  Constant2 : Constant  Value=Con_XPSbW_f32_1D100_UL
  Constant3 : Constant  Value=Con_XPSbW_f32_Zero_UL
  Signal Copy3 : SignalConversion  OverrideOpt=off
  SignalValidityJudgementFloat4 : XpengCHASbWLib/XpengCHASbWAlgoLib/Diagnostic/SignalValidityJudgementFloat
      settings: SourceProductName=Xpeng CHA SbW Lib
  Switch : XpengCHASbWLib/XpengCHASbWBaseLib/Signal Routing/Switch  Criteria=u2 ~= 0  Threshold=0  InputSameDT=on  OutMin=[]  OutMax=[]  SaturateOnIntegerOverflow=on  SampleTime=-1  AllowDiffInputSizes=off
      settings: AttributesFormatString=%<Criteria>  SourceProductName=Xpeng CHA SbW Lib
  f32_MotAgArbd_deg : Outport
  wires:
  Constant1/1 -> SignalValidityJudgementFloat4/3
  ES003_f32_MotAgArbd_deg_gdf32_read/1 -> Signal Copy3/1, SignalValidityJudgementFloat4/1
  Constant2/1 -> SignalValidityJudgementFloat4/4
  Switch/1 -> f32_MotAgArbd_deg/1
  Signal Copy3/1 -> Switch/1
  SignalValidityJudgementFloat4/1 -> Switch/2
  Constant3/1 -> Switch/3
  Constant/1 -> SignalValidityJudgementFloat4/2

== system MF007_MotVltgSVPWM/MotVltgSVPWMPer1/SignalProcg/MotBrdgVltgCalc ==
  note: Description:
      | 1.XP版权；
  ES008_f32_MotBrdgVltg_V_gdf32_read : Inport
  Constant : Constant  Value=Con_XPSbW_f32_ES008EPSSupplyVltgMax_V
  Constant1 : Constant  Value=Con_XPSbW_f32_ES008EPSSupplyVltgMin_V
  Constant10 : Constant  Value=Con_XPSbW_b_True_UL  OutDataTypeStr=single
  Constant2 : Constant  Value=Con_XPSbW_f32_1D100_UL
  Constant3 : Constant  Value=CalC_MF007_f32_MotBrdgVltg_V
  Constant9 : Constant  Value=CalC_MF007_f32_BrdgVoltFbkFilCoeff_UL  OutDataTypeStr=single
  LPF_1stOrder_TypeK : XpengCHASbWLib/XpengCHASbWAlgoLib/Digital Filters/LPF_1stOrder_TypeK
      settings: SourceProductName=Xpeng CHA SbW Lib
  Signal Copy3 : SignalConversion  OverrideOpt=off
  SignalValidityJudgementFloat4 : XpengCHASbWLib/XpengCHASbWAlgoLib/Diagnostic/SignalValidityJudgementFloat
      settings: SourceProductName=Xpeng CHA SbW Lib
  Switch : XpengCHASbWLib/XpengCHASbWBaseLib/Signal Routing/Switch  Criteria=u2 ~= 0  Threshold=0  InputSameDT=on  OutMin=[]  OutMax=[]  SaturateOnIntegerOverflow=on  SampleTime=-1  AllowDiffInputSizes=off
      settings: AttributesFormatString=%<Criteria>  SourceProductName=Xpeng CHA SbW Lib
  f32_MotBrdgVltg_V : Outport
  wires:
  Constant1/1 -> SignalValidityJudgementFloat4/3
  ES008_f32_MotBrdgVltg_V_gdf32_read/1 -> Signal Copy3/1, SignalValidityJudgementFloat4/1
  Constant2/1 -> SignalValidityJudgementFloat4/4
  LPF_1stOrder_TypeK/1 -> f32_MotBrdgVltg_V/1
  Signal Copy3/1 -> Switch/1
  SignalValidityJudgementFloat4/1 -> Switch/2
  Constant3/1 -> Switch/3
  Constant/1 -> SignalValidityJudgementFloat4/2
  Constant10/1 -> LPF_1stOrder_TypeK/3
  Constant9/1 -> LPF_1stOrder_TypeK/2
  Switch/1 -> LPF_1stOrder_TypeK/1

== system MF007_MotVltgSVPWM/MotVltgSVPWMPer1/SignalProcg/MotCtrlModeCalc ==
  note: Description:
      | 1.XP版权；
  MF014_u8_MotCtrlMode_UL_gdu8_read : Inport
  Signal Copy6 : SignalConversion  OverrideOpt=off
  u8_MotCtrlMode_UL : Outport
  wires:
  Signal Copy6/1 -> u8_MotCtrlMode_UL/1
  MF014_u8_MotCtrlMode_UL_gdu8_read/1 -> Signal Copy6/1

== system MF007_MotVltgSVPWM/MotVltgSVPWMPer1/SignalProcg/MotCtrlVltgDAxisCmdCalc ==
  note: Description:
      | 1.XP版权；
  MF006_f32_MotCtrlVltgDAxisCmd_V_gdf32_read : Inport
  Signal Copy6 : SignalConversion  OverrideOpt=off
  f32_MotCtrlVltgDAxisCmd_V : Outport
  wires:
  Signal Copy6/1 -> f32_MotCtrlVltgDAxisCmd_V/1
  MF006_f32_MotCtrlVltgDAxisCmd_V_gdf32_read/1 -> Signal Copy6/1

== system MF007_MotVltgSVPWM/MotVltgSVPWMPer1/SignalProcg/MotCtrlVltgQAxisCmdCalc ==
  note: Description:
      | 1.XP版权；
  MF006_f32_MotCtrlVltgQAxisCmd_V_gdf32_read : Inport
  Signal Copy6 : SignalConversion  OverrideOpt=off
  f32_MotCtrlVltgQAxisCmd_V : Outport
  wires:
  Signal Copy6/1 -> f32_MotCtrlVltgQAxisCmd_V/1
  MF006_f32_MotCtrlVltgQAxisCmd_V_gdf32_read/1 -> Signal Copy6/1

== system MF007_MotVltgSVPWM/MotVltgSVPWMPer1/SignalProcg/MotVFCtrlVltgAlphaCalc ==
  note: Description:
      | 1.XP版权；
  MF011_f32_MotVFCtrlVltgAlpha_V_gdf32_read : Inport
  Signal Copy6 : SignalConversion  OverrideOpt=off
  f32_MotVFCtrlVltgAlpha_V : Outport
  wires:
  Signal Copy6/1 -> f32_MotVFCtrlVltgAlpha_V/1
  MF011_f32_MotVFCtrlVltgAlpha_V_gdf32_read/1 -> Signal Copy6/1

== system MF007_MotVltgSVPWM/MotVltgSVPWMPer1/SignalProcg/MotVFCtrlVltgBetaCalc ==
  note: Description:
      | 1.XP版权；
  MF011_f32_MotVFCtrlVltgBeta_V_gdf32_read : Inport
  Signal Copy6 : SignalConversion  OverrideOpt=off
  f32_MotVFCtrlVltgBeta_V : Outport
  wires:
  Signal Copy6/1 -> f32_MotVFCtrlVltgBeta_V/1
  MF011_f32_MotVFCtrlVltgBeta_V_gdf32_read/1 -> Signal Copy6/1

== system MF007_MotVltgSVPWM/MotVltgSVPWMPer1/SignalProcg/MotVelElecFildCalc ==
  note: Description:
      | 1.XP版权；
  ES004_f32_MotVelElecFild_radps_gdf32_read : Inport
  Constant4 : Constant  Value=Con_XPSbW_f32_ES004MotVelElecFildMax_radps
  Constant5 : Constant  Value=Con_XPSbW_f32_ES004MotVelElecFildMin_radps
  Constant6 : Constant  Value=Con_XPSbW_f32_1D100_UL
  Constant7 : Constant  Value=Con_XPSbW_f32_Zero_UL
  Signal Copy6 : SignalConversion  OverrideOpt=off
  SignalValidityJudgementFloat1 : XpengCHASbWLib/XpengCHASbWAlgoLib/Diagnostic/SignalValidityJudgementFloat
      settings: SourceProductName=Xpeng CHA SbW Lib
  Switch1 : XpengCHASbWLib/XpengCHASbWBaseLib/Signal Routing/Switch  Criteria=u2 ~= 0  Threshold=0  InputSameDT=on  OutMin=[]  OutMax=[]  SaturateOnIntegerOverflow=on  SampleTime=-1  AllowDiffInputSizes=off
      settings: AttributesFormatString=%<Criteria>  SourceProductName=Xpeng CHA SbW Lib
  f32_MotVelElecFild_radps : Outport
  wires:
  Constant6/1 -> SignalValidityJudgementFloat1/4
  Switch1/1 -> f32_MotVelElecFild_radps/1
  Constant7/1 -> Switch1/3
  ES004_f32_MotVelElecFild_radps_gdf32_read/1 -> Signal Copy6/1, SignalValidityJudgementFloat1/1
  Signal Copy6/1 -> Switch1/1
  Constant5/1 -> SignalValidityJudgementFloat1/3
  SignalValidityJudgementFloat1/1 -> Switch1/2
  Constant4/1 -> SignalValidityJudgementFloat1/2

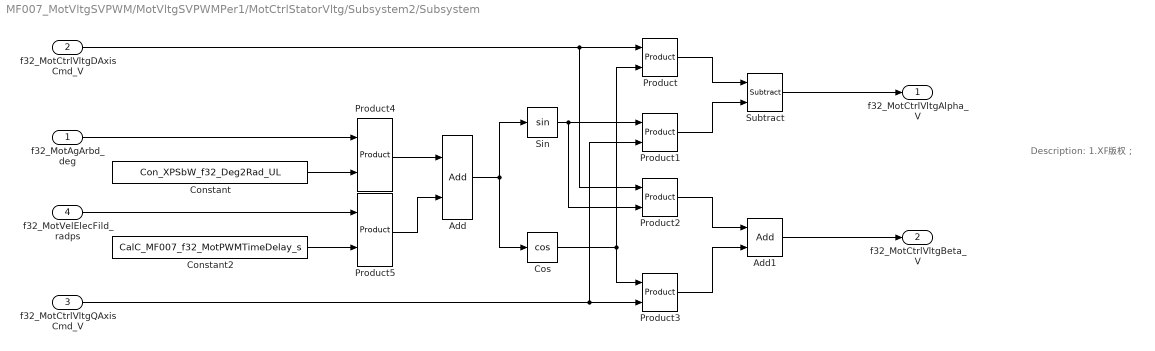
== system MF007_MotVltgSVPWM/MotVltgSVPWMPer1/MotCtrlStatorVltg/Subsystem2/Subsystem ==
  note: Description:
      | 1.XP版权；
  f32_MotAgArbd_deg : Inport
  f32_MotCtrlVltgDAxisCmd_V : Inport  Port=2
  f32_MotCtrlVltgQAxisCmd_V : Inport  Port=3
  f32_MotVelElecFild_radps : Inport  Port=4
  Add : XpengCHASbWLib/XpengCHASbWBaseLib/Math Operations/Add  Inputs=++  CollapseDim=1  OutMin=[]  OutMax=[]  SampleTime=-1
      settings: SourceProductName=Xpeng CHA SbW Lib
  Add1 : XpengCHASbWLib/XpengCHASbWBaseLib/Math Operations/Add  Inputs=++  CollapseDim=1  OutMin=[]  OutMax=[]  SampleTime=-1
      settings: SourceProductName=Xpeng CHA SbW Lib
  Constant : Constant  Value=Con_XPSbW_f32_Deg2Rad_UL
  Constant2 : Constant  Value=CalC_MF007_f32_MotPWMTimeDelay_s
  Cos : Trigonometry  Operator=cos
  Product{,1..5} (6 alike) : XpengCHASbWLib/XpengCHASbWBaseLib/Math Operations/Product  Inputs=2  Multiplication=Element-wise(.*)  CollapseDim=1  OutMin=[]  OutMax=[]  RndMeth=Zero  SaturateOnIntegerOverflow=on  SampleTime=-1
      settings: SourceProductName=Xpeng CHA SbW Lib
  Sin : Trigonometry
  Subtract : XpengCHASbWLib/XpengCHASbWBaseLib/Math Operations/Subtract  Inputs=+-  CollapseDim=1  OutMin=[]  OutMax=[]  SampleTime=-1
      settings: SourceProductName=Xpeng CHA SbW Lib
  f32_MotCtrlVltgAlpha_V : Outport
  f32_MotCtrlVltgBeta_V : Outport  Port=2
  wires:
  Product2/1 -> Add1/1
  f32_MotCtrlVltgQAxisCmd_V/1 -> Product1/2, Product3/2
  Product1/1 -> Subtract/2
  Product3/1 -> Add1/2
  Subtract/1 -> f32_MotCtrlVltgAlpha_V/1
  f32_MotCtrlVltgDAxisCmd_V/1 -> Product2/1, Product/1
  Cos/1 -> Product3/1, Product/2
  Product/1 -> Subtract/1
  Constant/1 -> Product4/2
  f32_MotVelElecFild_radps/1 -> Product5/1
  Add/1 -> Sin/1, Cos/1
  Product5/1 -> Add/2
  Sin/1 -> Product1/1, Product2/2
  f32_MotAgArbd_deg/1 -> Product4/1
  Add1/1 -> f32_MotCtrlVltgBeta_V/1
  Product4/1 -> Add/1
  Constant2/1 -> Product5/2

== system MF007_MotVltgSVPWM/MotVltgSVPWMPer1/MotCtrlStatorVltg/Subsystem2/Subsystem1 ==
  note: Description:
      | 1.XP版权；
  Constant18 : Constant  Value=CalC_XPSbW_b_MotTypSeln_UL
  If1 : XpengCHASbWLib/XpengCHASbWBaseLib/Ports&Subsystems/If  NumInputs=1  IfExpression=u1 == 0  ShowElse=on  SampleTime=-1
      settings: SourceProductName=Xpeng CHA SbW Lib
  StarMotor : Outport
  DeltaMotor : Outport  Port=2
  wires:
  Constant18/1 -> If1/1
  If1/1 -> StarMotor/1
  If1/2 -> DeltaMotor/1

== system MF007_MotVltgSVPWM/MotVltgSVPWMPer1/MotCtrlStatorVltg/Subsystem2/Subsystem2 ==
  note: Description:
      | 1.XP版权；
  f32_MotCtrlVltgAlphaRaw_V : Inport
  f32_MotCtrlVltgBetaRaw_V : Inport  Port=2
  StarMotor : ActionPort  ActionPortLabel=if(u1 == 0)
  Signal Copy : SignalConversion  OverrideOpt=off
  Signal Copy1 : SignalConversion  OverrideOpt=off
  f32_StarMotCtrlVltgAlpha_V : Outport
  f32_StarMotCtrlVltgBeta_V : Outport  Port=2
  wires:
  f32_MotCtrlVltgAlphaRaw_V/1 -> Signal Copy/1
  f32_MotCtrlVltgBetaRaw_V/1 -> Signal Copy1/1
  Signal Copy/1 -> f32_StarMotCtrlVltgAlpha_V/1
  Signal Copy1/1 -> f32_StarMotCtrlVltgBeta_V/1

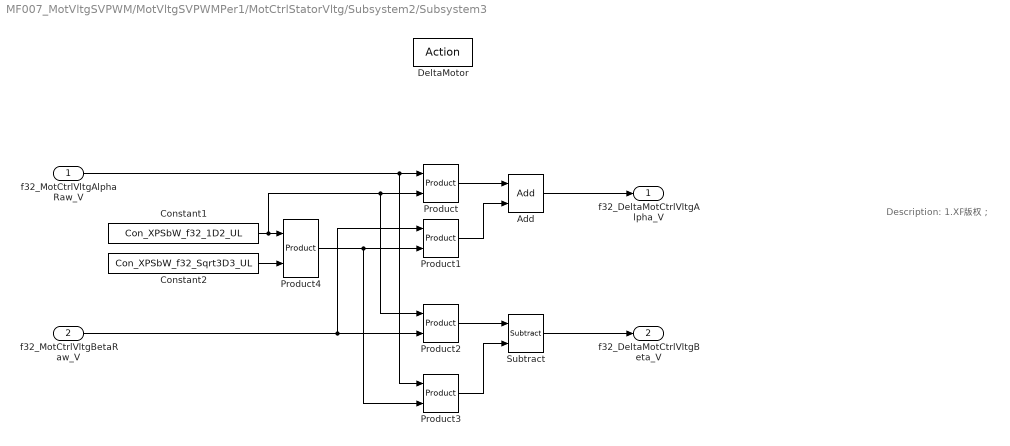
== system MF007_MotVltgSVPWM/MotVltgSVPWMPer1/MotCtrlStatorVltg/Subsystem2/Subsystem3 ==
  note: Description:
      | 1.XP版权；
  f32_MotCtrlVltgAlphaRaw_V : Inport
  f32_MotCtrlVltgBetaRaw_V : Inport  Port=2
  DeltaMotor : ActionPort  ActionPortLabel=else
  Add : XpengCHASbWLib/XpengCHASbWBaseLib/Math Operations/Add  Inputs=++  CollapseDim=1  OutMin=[]  OutMax=[]  SampleTime=-1
      settings: SourceProductName=Xpeng CHA SbW Lib
  Constant1 : Constant  Value=Con_XPSbW_f32_1D2_UL  OutDataTypeStr=single
  Constant2 : Constant  Value=Con_XPSbW_f32_Sqrt3D3_UL  OutDataTypeStr=single
  Product{,1..4} (5 alike) : XpengCHASbWLib/XpengCHASbWBaseLib/Math Operations/Product  Inputs=2  Multiplication=Element-wise(.*)  CollapseDim=1  OutMin=[]  OutMax=[]  RndMeth=Zero  SaturateOnIntegerOverflow=on  SampleTime=-1
      settings: SourceProductName=Xpeng CHA SbW Lib
  Subtract : XpengCHASbWLib/XpengCHASbWBaseLib/Math Operations/Subtract  Inputs=+-  CollapseDim=1  OutMin=[]  OutMax=[]  SampleTime=-1
      settings: SourceProductName=Xpeng CHA SbW Lib
  f32_DeltaMotCtrlVltgAlpha_V : Outport
  f32_DeltaMotCtrlVltgBeta_V : Outport  Port=2
  wires:
  f32_MotCtrlVltgAlphaRaw_V/1 -> Product3/1, Product/1
  Subtract/1 -> f32_DeltaMotCtrlVltgBeta_V/1
  Add/1 -> f32_DeltaMotCtrlVltgAlpha_V/1
  Product/1 -> Add/1
  Product1/1 -> Add/2
  f32_MotCtrlVltgBetaRaw_V/1 -> Product1/1, Product2/2
  Constant1/1 -> Product2/1, Product/2, Product4/1
  Constant2/1 -> Product4/2
  Product4/1 -> Product3/2, Product1/2
  Product2/1 -> Subtract/1
  Product3/1 -> Subtract/2

== system MF007_MotVltgSVPWM/MotVltgSVPWMPer1/MotCtrlStatorVltg/Subsystem2/Subsystem4 ==
  note: Description:
      | 1.XP版权；
  f32_StarMotCtrlVltgAlpha_V : Inport
  f32_StarMotCtrlVltgBeta_V : Inport  Port=2
  f32_DeltaMotCtrlVltgAlpha_V : Inport  Port=3
  f32_DeltaMotCtrlVltgBeta_V : Inport  Port=4
  Merge : Merge
  Merge1 : Merge
  f32_MotCtrlVltgAlphaRaw_V : Outport
  f32_MotCtrlVltgBetaRaw_V : Outport  Port=2
  wires:
  f32_StarMotCtrlVltgAlpha_V/1 -> Merge/1
  f32_DeltaMotCtrlVltgAlpha_V/1 -> Merge/2
  Merge/1 -> f32_MotCtrlVltgAlphaRaw_V/1
  f32_StarMotCtrlVltgBeta_V/1 -> Merge1/1
  f32_DeltaMotCtrlVltgBeta_V/1 -> Merge1/2
  Merge1/1 -> f32_MotCtrlVltgBetaRaw_V/1
